simulink model "laba3"  (Simulink 7.0)
settings: Solver=ode45  StartTime=0.0  StopTime=45.0  RelTol=1e-3
settings Model: Creator=liz  LastModifiedBy=liz

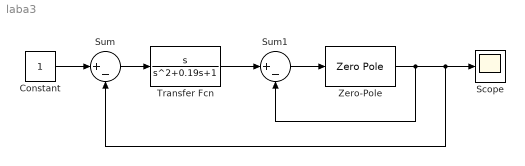
== system laba3 ==
  Constant : Constant  OutDataType=sfix(16)  OutScaling=2^0
  Scope : Scope
  Sum : Sum  Inputs=|+-  OutDataType=sfix(16)  OutScaling=2^0
  Sum1 : Sum  Inputs=|+-  OutDataType=sfix(16)  OutScaling=2^0
  Transfer Fcn : TransferFcn  Numerator=[1 0]  Denominator=[1 0.19 1]
  Zero-Pole : ZeroPole  Zeros=[0]  Poles=[-0.05 -1]
  wires:
  Constant/1 -> Sum/1
  Sum/1 -> Transfer Fcn/1
  Transfer Fcn/1 -> Sum1/1
  Sum1/1 -> Zero-Pole/1
  Zero-Pole/1 -> Sum/2, Scope/1, Sum1/2
